simulink model "Assignement_Simulink_2"  (R2022b)
settings: Solver=ode8  StartTime=0.0  StopTime=20000  FixedStep=0.1  RelTol=1e-3
values from neighbouring files (symbols this model uses):
  a = 6.943e6    (= 6943000)    [Assignement_Script.m]
  A0 = eye(3,3)    [Assignement_Script.m]
  A1 = 0.02    [Assignement_Script.m]
  A2 = A1    (= 0.02)    [Assignement_Script.m]
  A3 = A1    (= 0.02)    [Assignement_Script.m]
  alpha_1 = 0.5    [Assignement_Script.m]
  alpha_2 = 0.5    [Assignement_Script.m]
  C_d = 2.1    [Assignement_Script.m]
  e = 0    [Assignement_Script.m]
  epsilon = 0.4093    [Assignement_Script.m]
  G = 6.6743e-11    [Assignement_Script.m]
  H0 = sqrt(g_10^2+g_11^2+h_11^2)    [Assignement_Script.m]
  i = 0.8    [Assignement_Script.m]
  I = 10^-2*diag([100.9,25.1,91.6])    [Assignement_Script.m]
  j_B = [0.01;0.05;0.01]    [Assignement_Script.m]
  k_d_detumbling = 0.01    [Assignement_Script.m]
  k_d_nadir = 0.012    [Assignement_Script.m]
  k_p_nadir = 0.012    [Assignement_Script.m]
  M_Earth = 5.972e24    (= 5.972e+24)    [Assignement_Script.m]
  n = sqrt(G*M_Earth/a^3)    [Assignement_Script.m]
  n_sun = 2*pi/T_sun    (= 1.99238499086e-07)    [Assignement_Script.m]
  omega_detumbling = [0; 0; n_SC]    [Assignement_Script.m]
  omega_nadir = omega_detumbling    [Assignement_Script.m]
  P = F_e/c    (= 4.52666666667e-06)    [Assignement_Script.m]
  position = 1e-2*[10,0,0;0,10,0;-10,0,0;0,-10,0;0,0,15;                                     0,0,-15;0,45,0;0,45,0;0,-45,0;0,-45,0]    [Assignement_Script.m]
  R_Earth = 6.378e6    (= 6378000)    [Assignement_Script.m]
  R_sun = 149597870000    [Assignement_Script.m]
  rhoD_vector = ones(10,1)*0.1    [Assignement_Script.m]
  rhoS_vector = ones(10,1)*0.5    [Assignement_Script.m]
  Surfaces_Matrix = [6e-2;6e-2;6e-2;6e-2;4e-2;4e-2;12e-2;                                                     12e-2;12e-2;12e-2]    [Assignement_Script.m]
  theta0 = 0    [Assignement_Script.m]
  Theta_m = deg2rad(11.5)    [Assignement_Script.m]
  time_detumbling = 500    [Assignement_Script.m]
  time_nadir_pointing = 500    [Assignement_Script.m]
  Versor_Surfaces_Matrix = [  1 , 0 ,-1 , 0 , 0 , 0 , 1 ,-1 , 1 ,-1 ... (first row only)    [Assignement_Script.m]
  w0 = [0.01;0.01;0.2]    [Assignement_Script.m]
  w_Earth = 7.29e-5    (= 7.29e-05)    [Assignement_Script.m]
undefined symbols (not defined in the file or in its folder): Gyroscope, HS, k_d_slew, k_i_tracking, k_p_slew, omega_slew, RW, SunSensor, time_slew
libraries: simulink_extras x14, sharedutil x12, vrlib x11, matrix_library x11, sharedtransform x2
(part 3 of 3)

== matlab function Assignement_Simulink_2/Subsystem2/Algebraic method/MATLAB Function ==
  data: A input; x output; x0 input
function x  = eigpower_io(A, x0)
tol = 1e-4;
y = x0/norm(x0);  % approssimazione autovettore
lambda = y'*A*y; % approssiamzione autovalore
lambda_ex = lambda;
x = A*y;
y = x/norm(x);
lambda = y'*A*y;

while (abs(lambda-lambda_ex)/abs(lambda))>tol
    lambda_ex = lambda;
    x = A*y;
    y = x/norm(x);
    lambda = y'*A*y;
end

end

== matlab function Assignement_Simulink_2/Subsystem2/Algebraic method/MATLAB Function1 ==
  data: q input; DCM output
function DCM = fcn(q)

q1 = q(1);
q2 = q(2);
q3 = q(3);
q4 = q(4);

DCM = [q1^2-q2^2-q3^2+q4^2, 2*(q1*q2+q3*q4), 2*(q1*q3-q2*q4);
        2*(q1*q2-q3*q4), -q1^2+q2^2-q3^2+q4^2, 2*(q2*q3+q1*q4);
        2*(q1*q3+q2*q4), 2*(q2*q3-q1*q4), -q1^2-q2^2+q3^2+q4^2];

end

== matlab function Assignement_Simulink_2/Subsystem2/Gyro propagation/Perpendicularity/MATLAB Function2 ==
  data: DCM input; perpendicularity_flag output
function perpendicularity_flag = fcn(DCM)
    

perpendicularity_flag =zeros(3,1);

    x   = DCM(1,:);
    y   = DCM(2,:);
    z   = DCM(3,:);

    perpendicularity_flag(1)=dot(x,y);
    perpendicularity_flag(2)=dot(x,z);
    perpendicularity_flag(3)=dot(z,y);

end
